simulink model "mpc_SuboptimalSolution"  (R2023a)
settings: Solver=VariableStepAuto  StartTime=0.0  StopTime=T  RelTol=1e-3
values from neighbouring files (symbols this model uses):
  nOV = 3    [UseSuboptimalSolutionInFastMPC1.m]
  Ts = 0.1    [UseSuboptimalSolutionInFastMPC1.m]
libraries: cstblocks x2, mpclib x2, simulink x1
settings Model: Creator=The MathWorks, Inc.  LastModifiedBy=The MathWorks, Inc.
settings SolverCC: AlgebraicLoopSolver=TrustRegion
settings DataIOCC: ReturnWorkspaceOutputs=off
settings DebuggingCC: UnconnectedInputMsg=warning  UnconnectedOutputMsg=warning  UnconnectedLineMsg=warning  ArithmeticOperatorsInVariantConditions=warning
settings ModelReferenceCC: EnableRefExpFcnMdlSchedulingChecks=on
settings SFSimCC: SimUseLocalCustomCode=off  CustomCodeUndefinedFunction=UseInterfaceOnly
settings RTWCC: RTWUseLocalCustomCode=off  DLArmComputeVersion=19.05
settings CodeAppCC: StateflowObjectComments=on

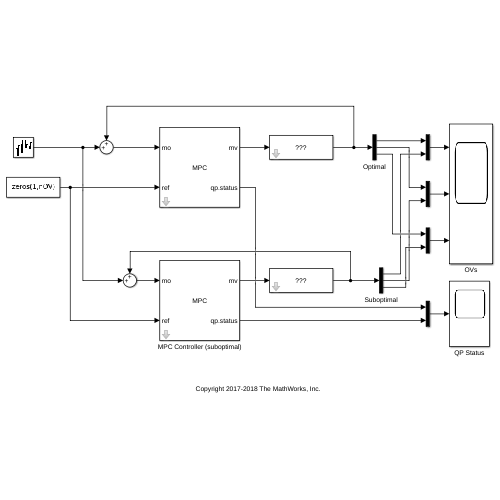
[thumbnail: Simulink's stored preview of the top-level diagram]
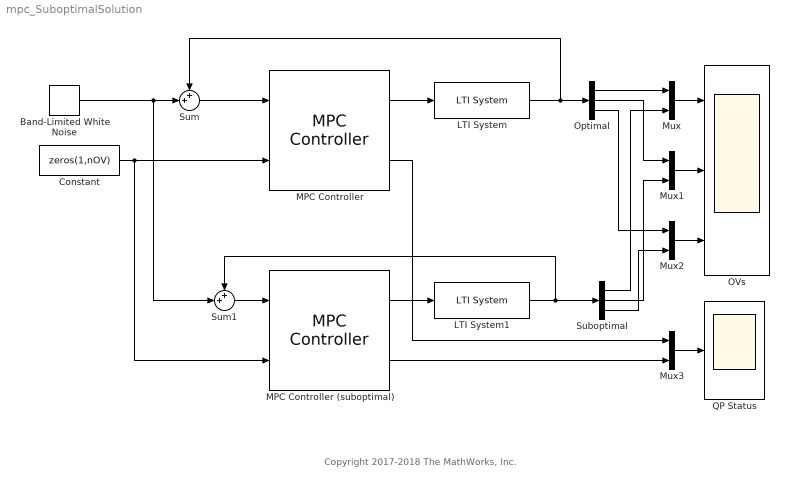
== system mpc_SuboptimalSolution ==
  note: Copyright 2017-2018 The MathWorks, Inc.
  Band-Limited White Noise : simulink/Sources/Band-Limited White Noise  Cov=5  Ts=Ts  seed=5687
  Constant : Constant  Value=zeros(1,nOV)
  LTI System : cstblocks/LTI System  sys=Plant  IC=[]
  LTI System1 : cstblocks/LTI System  sys=Plant  IC=[]
  MPC Controller : mpclib/MPC Controller  SCDEnableBlockLinearizationSpecification=on  mpcobj=mpcobj  is_multiple=0  enable_value=0  return_u0=off  updateMPCinCallerWorkspace=on  md_inport=off  mv_inport=off  uref_inport=off  return_cost=off  return_mvseq=off  return_qpstatus=on  return_xseq=off  return_state=off  return_ovseq=off  state_inport=off  umin_inport=off  umax_inport=off  ymin_inport=off  ymax_inport=off  cc_inport=off  ywt_inport=off  uwt_inport=off  duwt_inport=off  rhoeps_inport=off  pm_inport=off  MaximumP=10  HorizonChoice=FixedHorizon  n_ts=0.1  n_p=10  n_mv=3  n_md=0  n_ud=0  n_mo=3  n_uo=0  BlockDataType=double  SampleTimeInherited=off  switch_inport=off
  MPC Controller (suboptimal) : mpclib/MPC Controller  SCDEnableBlockLinearizationSpecification=on  mpcobj=mpcobjSub  is_multiple=0  enable_value=0  return_u0=off  updateMPCinCallerWorkspace=on  md_inport=off  mv_inport=off  uref_inport=off  return_cost=off  return_mvseq=off  return_qpstatus=on  return_xseq=off  return_state=off  return_ovseq=off  state_inport=off  umin_inport=off  umax_inport=off  ymin_inport=off  ymax_inport=off  cc_inport=off  ywt_inport=off  uwt_inport=off  duwt_inport=off  rhoeps_inport=off  pm_inport=off  MaximumP=10  HorizonChoice=FixedHorizon  n_ts=0.1  n_p=10  n_mv=3  n_md=0  n_ud=0  n_mo=3  n_uo=0  BlockDataType=double  SampleTimeInherited=off  switch_inport=off
  Mux{,1..3} (4 alike) : Mux  Inputs=2
  OVs : Scope  NumInputPorts=3
  Optimal : Demux  Outputs=3
  QP Status : Scope
  Suboptimal : Demux  Outputs=3
  Sum : Sum  Inputs=++|
  Sum1 : Sum  Inputs=++|
  wires:
  MPC Controller/1 -> LTI System/1
  Constant/1 -> MPC Controller/2, MPC Controller (suboptimal)/2
  Sum/1 -> MPC Controller/1
  LTI System/1 -> Optimal/1, Sum/1
  Band-Limited White Noise/1 -> Sum1/2, Sum/2
  MPC Controller (suboptimal)/1 -> LTI System1/1
  MPC Controller (suboptimal)/2 -> Mux3/2
  Sum1/1 -> MPC Controller (suboptimal)/1
  LTI System1/1 -> Sum1/1, Suboptimal/1
  Mux/1 -> OVs/1
  Mux1/1 -> OVs/2
  Mux2/1 -> OVs/3
  Optimal/1 -> Mux/1
  Optimal/2 -> Mux1/1
  Optimal/3 -> Mux2/1
  Suboptimal/1 -> Mux/2
  Suboptimal/2 -> Mux1/2
  Suboptimal/3 -> Mux2/2
  Mux3/1 -> QP Status/1
  MPC Controller/2 -> Mux3/1
